simulink model "example2019"  (R2019b)
settings: Solver=VariableStepAuto  StartTime=0.0  StopTime=stoptime  RelTol=1e-3
values from neighbouring files (symbols this model uses):
  A = [0 1;-5 -6]    [data.m]
  b = [0;1]    [data.m]
  ct = [10 1]    [data.m]
  x0 = [0.1;0]    [data.m]
settings Model: Creator=SURAJ  LastModifiedBy=sables
settings DataIOCC: ReturnWorkspaceOutputs=off
settings DebuggingCC: ArithmeticOperatorsInVariantConditions=warning
settings SFSimCC: SimUseLocalCustomCode=off  CustomCodeUndefinedFunction=UseInterfaceOnly
settings RTWCC: RTWUseLocalCustomCode=off

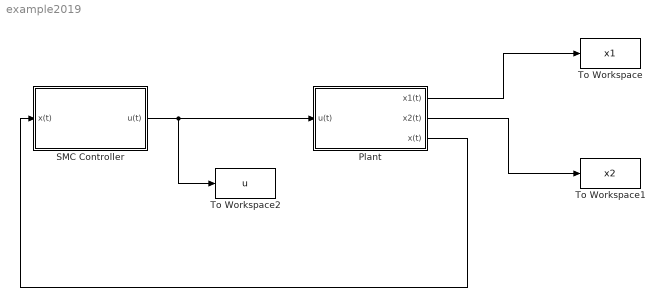
== system example2019 ==
  Plant : Subsystem
  SMC Controller : Subsystem
  To Workspace : ToWorkspace  VariableName=x1  SaveFormat=Timeseries  SampleTime=-1
  To Workspace1 : ToWorkspace  VariableName=x2  SaveFormat=Timeseries  SampleTime=-1
  To Workspace2 : ToWorkspace  VariableName=u  SaveFormat=Timeseries  SampleTime=-1
  wires:
  Plant/3(x(t)) -> SMC Controller/1(x(t))
  Plant/1(x1(t)) -> To Workspace/1
  Plant/2(x2(t)) -> To Workspace1/1
  SMC Controller/1(u(t)) -> To Workspace2/1, Plant/1(u(t))

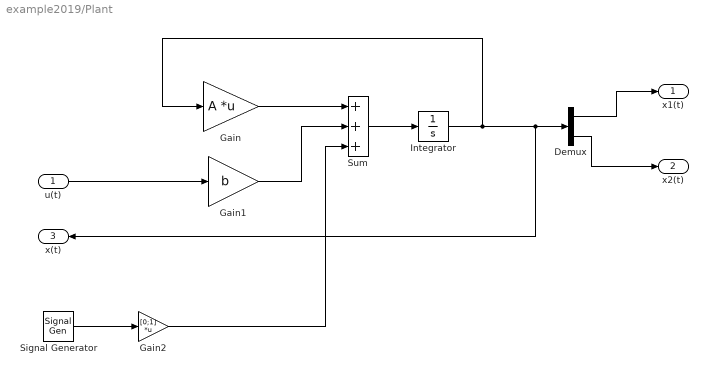
== system example2019/Plant ==
  u(t) : Inport
  Demux : Demux  Outputs=2
  Gain : Gain  Gain=A  Multiplication=Matrix(K*u) (u vector)
  Gain1 : Gain  Gain=b
  Gain2 : Gain  Gain=[0;1]  Multiplication=Matrix(K*u) (u vector)
  Integrator : Integrator  InitialCondition=x0
  Signal Generator : SignalGenerator  Frequency=0.1  Units=rad/sec
  Sum : Sum  Inputs=+++
  x1(t) : Outport  VectorParamsAs1DForOutWhenUnconnected=off
  x2(t) : Outport  Port=2  VectorParamsAs1DForOutWhenUnconnected=off
  x(t) : Outport  Port=3  VectorParamsAs1DForOutWhenUnconnected=off
  wires:
  Demux/1 -> x1(t)/1
  u(t)/1 -> Gain1/1
  Demux/2 -> x2(t)/1
  Gain1/1 -> Sum/2
  Integrator/1 -> Gain/1, x(t)/1, Demux/1
  Gain/1 -> Sum/1
  Sum/1 -> Integrator/1
  Signal Generator/1 -> Gain2/1
  Gain2/1 -> Sum/3

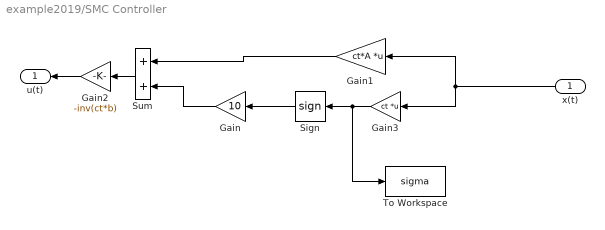
== system example2019/SMC Controller ==
  x(t) : Inport
  Gain : Gain  Gain=10
  Gain1 : Gain  Gain=ct*A  Multiplication=Matrix(K*u) (u vector)
  Gain2 : Gain  Gain=-inv(ct*b)
  Gain3 : Gain  Gain=ct  Multiplication=Matrix(K*u) (u vector)
  Sign : Signum  ZeroCross=off
  Sum : Sum
  To Workspace : ToWorkspace  VariableName=sigma  SaveFormat=Timeseries  SampleTime=-1
  u(t) : Outport  VectorParamsAs1DForOutWhenUnconnected=off
  wires:
  Gain2/1 -> u(t)/1
  Gain/1 -> Sum/2
  Sum/1 -> Gain2/1
  Sign/1 -> Gain/1
  Gain1/1 -> Sum/1
  Gain3/1 -> Sign/1, To Workspace/1
  x(t)/1 -> Gain1/1, Gain3/1
